simulink model "sFunctionTest"  (R2017b)
settings: Solver=ode5  StartTime=0.0  StopTime=2592000  FixedStep=0.0025  RelTol=1e-3
settings Model: Creator=davidlaredorazo  LastModifiedBy=davidlaredorazo

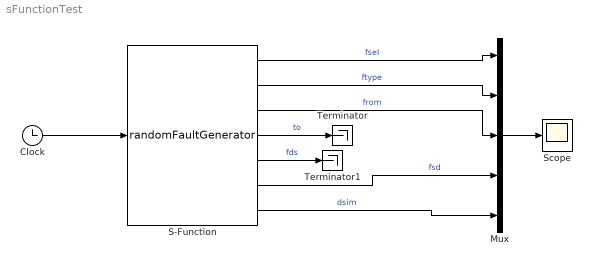
== system sFunctionTest ==
  Clock : Clock
  Mux : Mux  Inputs=5
  S-Function : S-Function  FunctionName=randomFaultGenerator  SFunctionDeploymentMode=off  EnableBusSupport=off
  Scope : Scope
  Terminator : Terminator
  Terminator1 : Terminator
  wires:
  S-Function/7 -> Mux/5  "dsim"
  Clock/1 -> S-Function/1
  S-Function/1 -> Mux/1  "fsel"
  S-Function/2 -> Mux/2  "ftype"
  S-Function/3 -> Mux/3  "from"
  S-Function/4 -> Terminator/1  "to"
  S-Function/5 -> Terminator1/1  "fds"
  S-Function/6 -> Mux/4  "fsd"
  Mux/1 -> Scope/1
